simulink subsystem "const_controller"  (R2024b)
settings: Solver=VariableStepAuto  StartTime=0.0  StopTime=10.0  RelTol=1e-3
undefined symbols (not defined in the file): brake_off, brake_on, const_brake
settings Model: Creator=yevge  LastModifiedBy=Aiden Gaydos

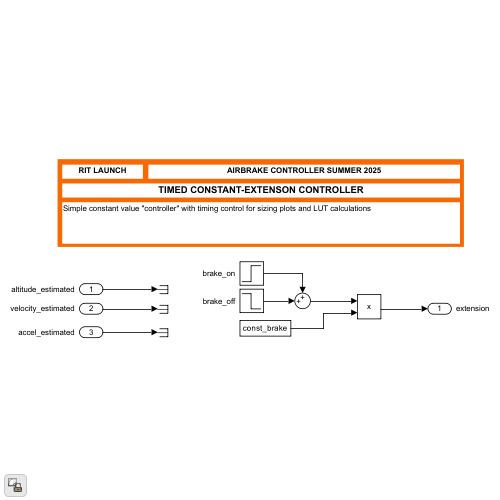
[thumbnail: Simulink's stored preview of the top-level diagram]
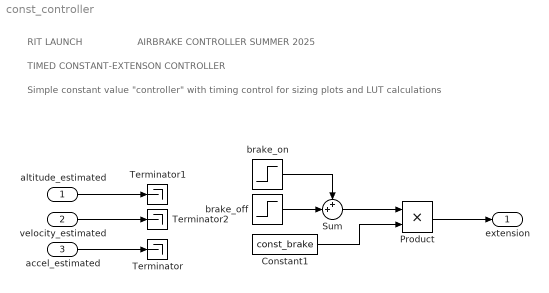
== system const_controller ==
  note: RIT LAUNCH
  note: AIRBRAKE CONTROLLER SUMMER 2025
  note: Simple constant value "controller" with timing control for sizing plots and LUT calculations
  note: TIMED CONSTANT-EXTENSON CONTROLLER
  altitude_estimated : Inport  Unit=m  PortDimensions=1
  velocity_estimated : Inport  Port=2  Unit=m/s  PortDimensions=1
  accel_estimated : Inport  Port=3  Unit=m/s^2  PortDimensions=1
  Constant1 : Constant  Value=const_brake
  Product : Product
  Sum : Sum  Inputs=++|
  Terminator : Terminator
  Terminator1 : Terminator
  Terminator2 : Terminator
  brake_off : Step  Time=brake_off  After=-1  SampleTime=0
  brake_on : Step  Time=brake_on  SampleTime=0
  extension : Outport  OutMin=0  OutMax=1  Unit=1  PortDimensions=1  InitialOutput=const_brake
  wires:
  accel_estimated/1 -> Terminator/1
  altitude_estimated/1 -> Terminator1/1
  velocity_estimated/1 -> Terminator2/1
  Constant1/1 -> Product/2
  brake_on/1 -> Sum/1
  brake_off/1 -> Sum/2
  Sum/1 -> Product/1
  Product/1 -> extension/1
